simulink library "FlatSatRead_lib"  (R2018b)
settings: Solver=VariableStepAuto  StartTime=0.0  StopTime=10.0  RelTol=1e-3
undefined symbols (not defined in the file or in its folder): mtq_dipole_body_Am2, rwa_torque_body_Nm
libraries: actuator_control_bus x1
settings Model: Creator=Taylor  LastModifiedBy=Taylor

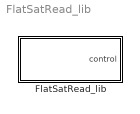
== system FlatSatRead_lib ==
  FlatSatRead_lib : Subsystem

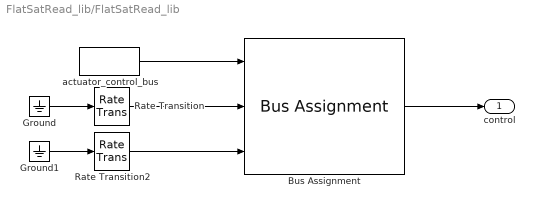
== system FlatSatRead_lib/FlatSatRead_lib ==
  Bus Assignment : BusAssignment  AssignedSignals=rwa_torque_body_Nm,mtq_dipole_body_Am2
  Ground : Ground
  Ground1 : Ground
  Rate Transition : RateTransition
  Rate Transition2 : RateTransition
  actuator_control_bus : actuator_control_bus/actuator_control_bus  SystemSampleTime=-1
  control : Outport  OutDataTypeStr=Bus: actuator_control
  wires:
  Rate Transition/1 -> Bus Assignment/2
  Ground1/1 -> Rate Transition2/1
  actuator_control_bus/1 -> Bus Assignment/1
  Rate Transition2/1 -> Bus Assignment/3
  Ground/1 -> Rate Transition/1
  Bus Assignment/1 -> control/1
